simulink model "Plant"  (R2016b)
settings: Solver=ode3  StartTime=0.0  StopTime=3000  RelTol=1e-3  EnableMultiTasking=on
PreLoadFcn:
  | fuz_sugeno5=readfis('fuz_sugeno5.fis');
StopFcn:
  | plot(h(:,1),h(:,2),'r',h(:,1),h(:,3),'b');grid;
  | xlabel('times');
  | ylabel('Muc nuoc bon 2');
  | legend('ref','measure',3);
libraries: fuzblock x1
settings Model: Creator=Administrator  LastModifiedBy=Truc
settings DataIOCC: LimitDataPoints=on  SaveFormat=Array
settings OptimizationCC: LifeSpan=inf
settings DebuggingCC: UnderspecifiedInitializationDetection=Classic  MergeDetectMultiDrivingBlocksExec=none  SolverPrmCheckMsg=warning  StateNameClashWarn=warning  SFUnexpectedBacktrackingDiag=warning  SFNoUnconditionalDefaultTransitionDiag=warning  SFExecutionAtInitializationDiag=none
settings HardwareCC: ProdBitPerPointer=32  ProdBitPerSizeT=32  ProdBitPerPtrDiffT=32  ProdLargestAtomicFloat=None  ProdIntDivRoundTo=Undefined  ProdEndianess=Unspecified  ProdWordSize=32  ProdHWDeviceType=32-bit Generic
settings ModelReferenceCC: PropagateSignalLabelsOutOfModel=off
settings GRTTargetCC: TargetLangStandard=C89/C90 (ANSI)  GeneratePreprocessorConditionals=Disable all
settings ConfigComp: CovMetricSettings=dw  CovHtmlReporting=on  CovSaveCumulativeToWorkspaceVar=on  CovSaveSingleToWorkspaceVar=on  CovExternalEMLEnable=off

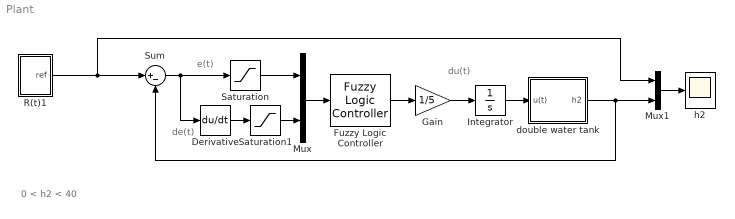
== system Plant ==
  note: du(t)
  note: e(t)
  note: de(t)
  note: 0 < h2 < 40
  Derivative : Derivative
  Fuzzy Logic Controller : fuzblock/Fuzzy Logic  Controller  fis=fuz_sugeno5
  Gain : Gain  Gain=1/5  SaturateOnIntegerOverflow=on  OutDataTypeStr=Inherit: Same as input  ParamDataTypeStr=Inherit: Same as input
  Integrator : Integrator  LimitOutput=on  UpperSaturationLimit=1  LowerSaturationLimit=0
  Mux : Mux  Inputs=2
  Mux1 : Mux  Inputs=2
  R(t)1 : Subsystem
  Saturation : Saturate  UpperLimit=20  LowerLimit=-20
  Saturation1 : Saturate  UpperLimit=1  LowerLimit=-1
  Sum : Sum  Inputs=|+-  SaturateOnIntegerOverflow=on
  double water tank : Subsystem  mask{k=600, A_1=300, A_2=300, a1=3, a2=2, g=981}
      mask prompts: A_1 "A1"; A_2 "A2"
  h2 : Scope
  wires:
  Mux/1 -> Fuzzy Logic Controller/1
  Sum/1 -> Derivative/1, Saturation/1
  Saturation/1 -> Mux/1
  Derivative/1 -> Saturation1/1
  Saturation1/1 -> Mux/2
  Integrator/1 -> double water tank/1(u(t))
  Fuzzy Logic Controller/1 -> Gain/1
  Gain/1 -> Integrator/1
  Mux1/1 -> h2/1
  double water tank/1(h2) -> Mux1/2, Sum/2
  R(t)1/1(ref) -> Sum/1, Mux1/1

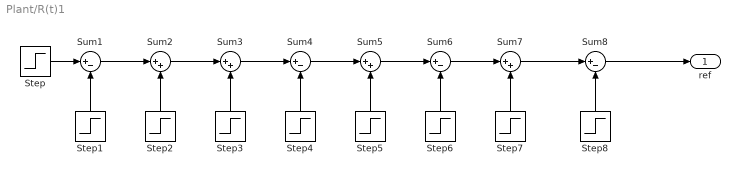
== system Plant/R(t)1 ==
  Step : Step  Time=0  After=15  SampleTime=0
  Step1 : Step  Time=250  After=5  SampleTime=0
  Step2 : Step  Time=500  After=5  SampleTime=0
  Step3 : Step  Time=750  After=15  SampleTime=0
  Step4 : Step  Time=1000  After=10  SampleTime=0
  Step5 : Step  Time=1250  After=15  SampleTime=0
  Step6 : Step  Time=1500  After=5  SampleTime=0
  Step7 : Step  Time=1750  After=10  SampleTime=0
  Step8 : Step  Time=2000  After=5  SampleTime=0
  Sum{1,4,6,8} (4 alike) : Sum  Inputs=|+-  SaturateOnIntegerOverflow=on
  Sum{2..3,5,7} (4 alike) : Sum  Inputs=|++  SaturateOnIntegerOverflow=on
  ref : Outport
  wires:
  Sum5/1 -> Sum6/1
  Step7/1 -> Sum7/2
  Sum6/1 -> Sum7/1
  Step6/1 -> Sum6/2
  Sum3/1 -> Sum4/1
  Step5/1 -> Sum5/2
  Sum4/1 -> Sum5/1
  Step4/1 -> Sum4/2
  Step3/1 -> Sum3/2
  Sum2/1 -> Sum3/1
  Step2/1 -> Sum2/2
  Sum1/1 -> Sum2/1
  Step1/1 -> Sum1/2
  Step/1 -> Sum1/1
  Step8/1 -> Sum8/2
  Sum8/1 -> ref/1
  Sum7/1 -> Sum8/1

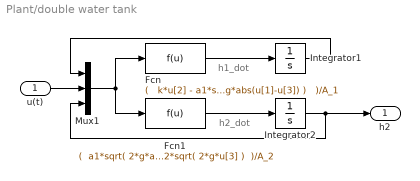
== system Plant/double water tank ==
  note: h1_dot
  note: h2_dot
  u(t) : Inport
  Fcn : Fcn  Expr="(   k*u[2] - a1*sqrt( 2*g*abs(u[1]-u[3]) )   )/A_1"
  Fcn1 : Fcn  Expr="(  a1*sqrt( 2*g*abs(u[1]-u[3]) ) - a2*sqrt( 2*g*u[3] )  )/A_2"
  Integrator1 : Integrator  LimitOutput=on  UpperSaturationLimit=100  LowerSaturationLimit=0
  Integrator2 : Integrator  LimitOutput=on  UpperSaturationLimit=100  LowerSaturationLimit=0
  Mux1 : Mux  Inputs=3
  h2 : Outport
  wires:
  u(t)/1 -> Mux1/2
  Integrator2/1 -> h2/1, Mux1/3
  Integrator1/1 -> Mux1/1
  Fcn/1 -> Integrator1/1
  Mux1/1 -> Fcn/1, Fcn1/1
  Fcn1/1 -> Integrator2/1
